simulink model "mse_model"  (R2025a)
settings: Solver=VariableStepAuto  StartTime=0.0  StopTime=100  RelTol=1e-3
values from neighbouring files (symbols this model uses):
  Gp = tf([1,5],[1,3,6])    [mse.m]
  Tf = 1    [gradient.m]    (also in mse.m)
settings Model: Creator=Korisnik  LastModifiedBy=Korisnik

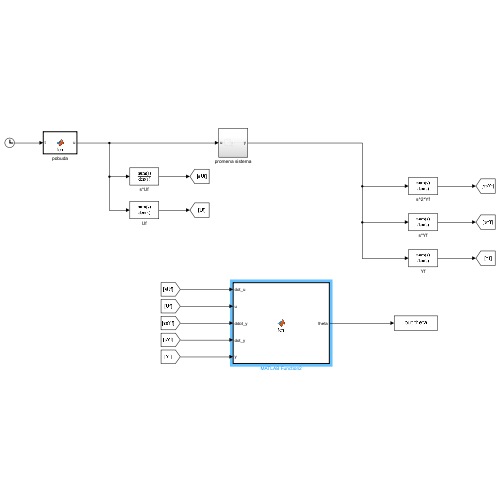
[thumbnail: Simulink's stored preview of the top-level diagram]
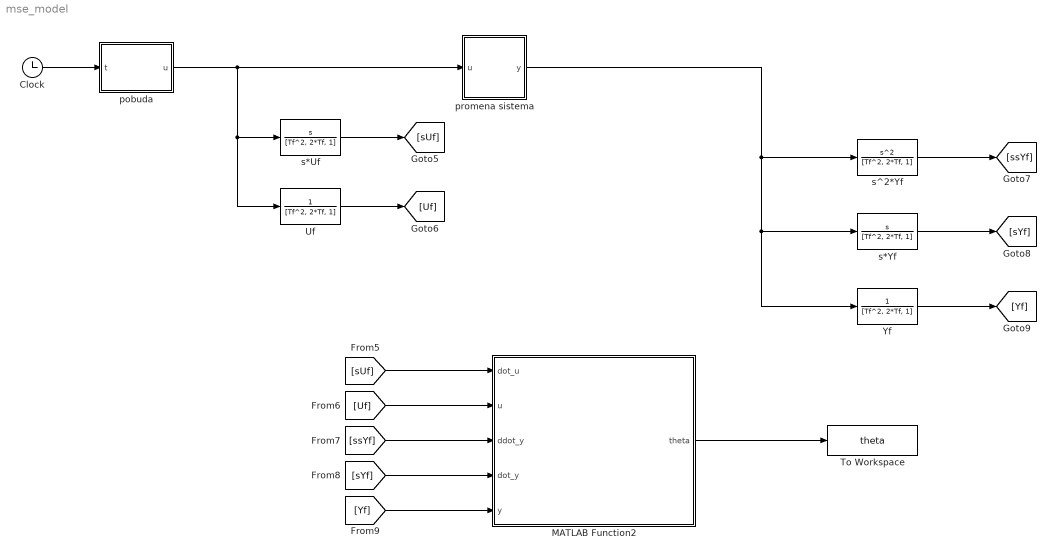
== system mse_model ==
  Clock : Clock
  MATLAB Function2 : MATLAB Function  TreatAsAtomicUnit=on
  To Workspace : ToWorkspace  VariableName=theta  SaveFormat=Timeseries  SampleTime=-1
  Uf : TransferFcn  Numerator=1  Denominator=[Tf^2, 2*Tf, 1]
  Yf : TransferFcn  Numerator=1  Denominator=[Tf^2, 2*Tf, 1]
  pobuda : MATLAB Function  TreatAsAtomicUnit=on
  promena sistema : Subsystem
  s*Uf : TransferFcn  Numerator=[1, 0]  Denominator=[Tf^2, 2*Tf, 1]
  s*Yf : TransferFcn  Numerator=[1, 0]  Denominator=[Tf^2, 2*Tf, 1]
  s^2*Yf : TransferFcn  Numerator=[1, 0, 0]  Denominator=[Tf^2, 2*Tf, 1]
  wires:
  [Yf] -> MATLAB Function2/5(y)
  Clock/1 -> pobuda/1(t)
  pobuda/1(u) -> Uf/1, s*Uf/1, promena sistema/1(u)
  [sYf] -> MATLAB Function2/4(dot_y)
  s*Yf/1 -> [sYf]
  [sUf] -> MATLAB Function2/1(dot_u)
  Yf/1 -> [Yf]
  Uf/1 -> [Uf]
  [ssYf] -> MATLAB Function2/3(ddot_y)
  s^2*Yf/1 -> [ssYf]
  s*Uf/1 -> [sUf]
  promena sistema/1(y) -> Yf/1, s*Yf/1, s^2*Yf/1
  MATLAB Function2/1(theta) -> To Workspace/1
  [Uf] -> MATLAB Function2/2(u)

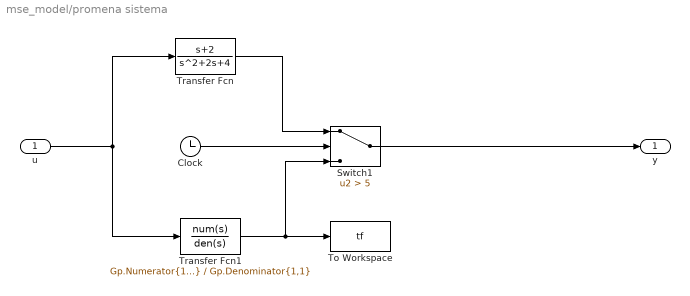
== system mse_model/promena sistema ==
  u : Inport
  Clock : Clock
      settings: Decimation=3
  Switch1 : Switch  Criteria=u2 > Threshold  Threshold=5  SaturateOnIntegerOverflow=off  InputSameDT=off
  To Workspace : ToWorkspace  VariableName=tf  SaveFormat=Timeseries  SampleTime=-1
  Transfer Fcn : TransferFcn  Numerator=[1, 2]  Denominator=[1, 2, 4]
  Transfer Fcn1 : TransferFcn  Numerator=Gp.Numerator{1,1}  Denominator=Gp.Denominator{1,1}
  y : Outport
  wires:
  Switch1/1 -> y/1
  u/1 -> Transfer Fcn1/1, Transfer Fcn/1
  Clock/1 -> Switch1/2
  Transfer Fcn/1 -> Switch1/1
  Transfer Fcn1/1 -> To Workspace/1, Switch1/3

== matlab function mse_model/pobuda ==
  data: t input; u output
function u = fcn(t)
    u = 0;
    fmax = 10;
    for i = 1:fmax
        u = u + sin(2 * pi * i * t);
    end

== matlab function mse_model/MATLAB Function2 ==
  settings: updateMethod=DISCRETE  sampleTime=0.01
  data: dot_u input; u input; theta output; ddot_y input; dot_y input; y input
% Kod sa casa
function theta = fcn(dot_u, u, ddot_y, dot_y, y)
    persistent P;
    persistent Theta;
    lambda = 0.999;
    
    phi = [-dot_y; -y; dot_u; u];
    eta = ddot_y;
    
    if isempty(Theta)
        Theta = zeros(length(phi), 1);
    end

    if isempty(P)
        P = 10000 * eye(length(phi), length(phi));
    end

    % P = 1 / lambda * (P - (P * (phi * phi') * P) / (lambda + phi' * P * phi));
    P = 1 / lambda * (P - (P * (phi * phi') * P) / (lambda + phi' * P * phi));
    
    Theta = Theta + P * phi * (eta - phi' * Theta);
    theta = Theta;
end
